simulink model "TestWalsh02_home"  (R2021a)
settings: Solver=VariableStepAuto  StartTime=0.0  StopTime=96  RelTol=1e-3
libraries: dspspect3 x4
settings Model: Creator=alexandr.lanin  LastModifiedBy=Alex
settings SolverCC: AlgebraicLoopSolver=TrustRegion
settings DataIOCC: ReturnWorkspaceOutputs=off
settings DebuggingCC: SFMachineParentedDataDiag=warning  ArithmeticOperatorsInVariantConditions=warning
settings SFSimCC: SimUseLocalCustomCode=off  CustomCodeUndefinedFunction=UseInterfaceOnly
settings RTWCC: RTWUseLocalCustomCode=off
settings CodeAppCC: StateflowObjectComments=on

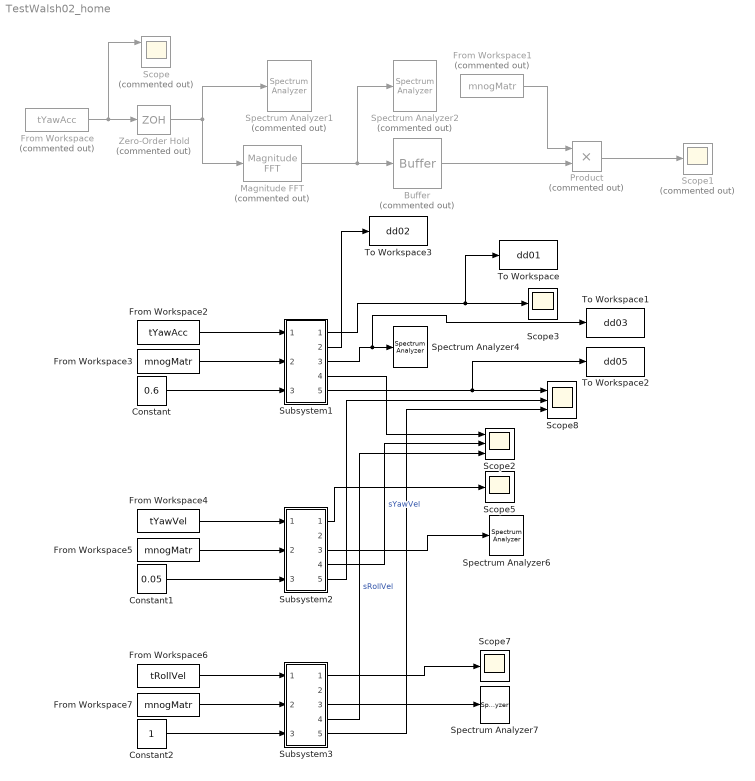
== system TestWalsh02_home ==
  Buffer : Buffer  Commented=on  OutputFrames=off
  Constant : Constant  Value=0.6
  Constant1 : Constant  Value=0.05
  Constant2 : Constant
  From Workspace : FromWorkspace  Commented=on  VariableName=tYawAcc
  From Workspace1 : FromWorkspace  Commented=on  VariableName=mnogMatr
  From Workspace2 : FromWorkspace  VariableName=tYawAcc
  From Workspace3 : FromWorkspace  VariableName=mnogMatr
  From Workspace4 : FromWorkspace  VariableName=tYawVel
  From Workspace5 : FromWorkspace  VariableName=mnogMatr
  From Workspace6 : FromWorkspace  VariableName=tRollVel
  From Workspace7 : FromWorkspace  VariableName=mnogMatr
  Magnitude FFT : dspspect3/Magnitude FFT  Commented=on  mag_or_magsq=Magnitude squared  FFTImplementation=Auto  fftLenInherit=off  fftsize=64  WrapInput=on
      settings: SourceProductBaseCode=DS
  Product : Product  Commented=on
  Scope : Scope  Commented=on  NumInputPorts=3
  Scope1 : Scope  Commented=on
  Scope2 : Scope  NumInputPorts=3
  Scope3 : Scope
  Scope5 : Scope
  Scope7 : Scope
  Scope8 : Scope  NumInputPorts=3
  Spectrum Analyzer1 : SpectrumAnalyzer  Commented=on
  Spectrum Analyzer2 : SpectrumAnalyzer  Commented=on
  Spectrum Analyzer4 : SpectrumAnalyzer
  Spectrum Analyzer6 : SpectrumAnalyzer
  Spectrum Analyzer7 : SpectrumAnalyzer
  Subsystem1 : Subsystem
  Subsystem2 : Subsystem
  Subsystem3 : Subsystem
  To Workspace : ToWorkspace  VariableName=dd01  SaveFormat=Timeseries  SampleTime=-1
  To Workspace1 : ToWorkspace  VariableName=dd03  SaveFormat=Timeseries  SampleTime=-1
  To Workspace2 : ToWorkspace  VariableName=dd05  SaveFormat=Timeseries  SampleTime=-1
  To Workspace3 : ToWorkspace  VariableName=dd02  SaveFormat=Timeseries  SampleTime=-1
  Zero-Order Hold : ZeroOrderHold  Commented=on  SampleTime=0.01
  wires:
  From Workspace/1 -> Zero-Order Hold/1, Scope/1
  Magnitude FFT/1 -> Buffer/1, Spectrum Analyzer2/1
  Zero-Order Hold/1 -> Magnitude FFT/1, Spectrum Analyzer1/1
  Buffer/1 -> Product/2
  From Workspace1/1 -> Product/1
  Product/1 -> Scope1/1
  From Workspace3/1 -> Subsystem1/2(In2)
  From Workspace2/1 -> Subsystem1/1(In1)
  Subsystem1/3(Out3) -> To Workspace1/1, Spectrum Analyzer4/1
  Subsystem1/1(Out1) -> To Workspace/1, Scope3/1
  Subsystem1/4(Out4) -> Scope2/1
  Subsystem2/1(Out1) -> Scope5/1
  Subsystem2/3(Out3) -> Spectrum Analyzer6/1
  From Workspace4/1 -> Subsystem2/1(In1)
  From Workspace5/1 -> Subsystem2/2(In2)
  Subsystem3/4(Out4) -> Scope2/3  "sRollVel"
  Subsystem3/1(Out1) -> Scope7/1
  From Workspace6/1 -> Subsystem3/1(In1)
  Subsystem3/3(Out3) -> Spectrum Analyzer7/1
  From Workspace7/1 -> Subsystem3/2(In3)
  Constant/1 -> Subsystem1/3(In3)
  Constant1/1 -> Subsystem2/3(In3)
  Constant2/1 -> Subsystem3/3(In2)
  Subsystem2/4(Out4) -> Scope2/2  "sYawVel"
  Subsystem3/5(Out5) -> Scope8/3
  Subsystem2/5(Out5) -> Scope8/2
  Subsystem1/5(Out5) -> To Workspace2/1, Scope8/1
  Subsystem1/2(Out2) -> To Workspace3/1

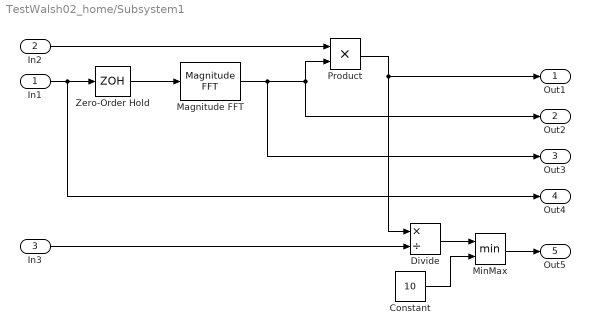
== system TestWalsh02_home/Subsystem1 ==
  In1 : Inport
  In2 : Inport  Port=2
  In3 : Inport  Port=3
  Constant : Constant  Value=10
  Divide : Product  Inputs=*/
  Magnitude FFT : dspspect3/Magnitude FFT  mag_or_magsq=Magnitude squared  FFTImplementation=Auto  fftLenInherit=off  fftsize=64  WrapInput=on
      settings: SourceProductBaseCode=DS
  MinMax : MinMax  Inputs=2
  Product : Product
  Zero-Order Hold : ZeroOrderHold  SampleTime=0.01
  Out1 : Outport
  Out2 : Outport  Port=2
  Out3 : Outport  Port=3
  Out4 : Outport  Port=4
  Out5 : Outport  Port=5
  wires:
  Zero-Order Hold/1 -> Magnitude FFT/1
  In1/1 -> Out4/1, Zero-Order Hold/1
  In2/1 -> Product/1
  In3/1 -> Divide/2
  Divide/1 -> MinMax/1
  Constant/1 -> MinMax/2
  MinMax/1 -> Out5/1
  Product/1 -> Divide/1, Out1/1
  Magnitude FFT/1 -> Out2/1, Product/2, Out3/1

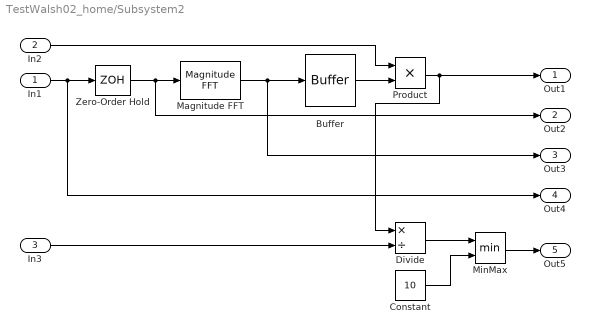
== system TestWalsh02_home/Subsystem2 ==
  In1 : Inport
  In2 : Inport  Port=2
  In3 : Inport  Port=3
  Buffer : Buffer  OutputFrames=off
  Constant : Constant  Value=10
  Divide : Product  Inputs=*/
  Magnitude FFT : dspspect3/Magnitude FFT  mag_or_magsq=Magnitude squared  FFTImplementation=Auto  fftLenInherit=off  fftsize=64  WrapInput=on
      settings: SourceProductBaseCode=DS
  MinMax : MinMax  Inputs=2
  Product : Product
  Zero-Order Hold : ZeroOrderHold  SampleTime=0.01
  Out1 : Outport
  Out2 : Outport  Port=2
  Out3 : Outport  Port=3
  Out4 : Outport  Port=4
  Out5 : Outport  Port=5
  wires:
  Zero-Order Hold/1 -> Out2/1, Magnitude FFT/1
  In1/1 -> Out4/1, Zero-Order Hold/1
  Magnitude FFT/1 -> Out3/1, Buffer/1
  Buffer/1 -> Product/2
  Product/1 -> Divide/1, Out1/1
  In2/1 -> Product/1
  In3/1 -> Divide/2
  Divide/1 -> MinMax/1
  Constant/1 -> MinMax/2
  MinMax/1 -> Out5/1

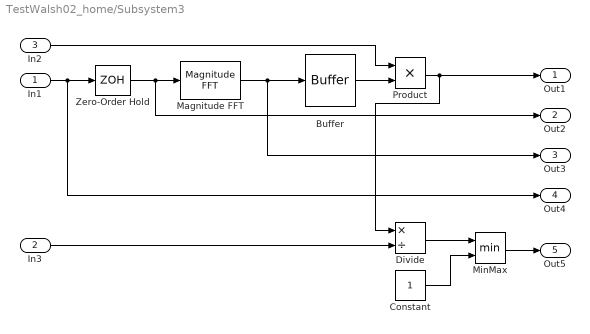
== system TestWalsh02_home/Subsystem3 ==
  In1 : Inport
  In3 : Inport  Port=2
  In2 : Inport  Port=3
  Buffer : Buffer  OutputFrames=off
  Constant : Constant
  Divide : Product  Inputs=*/
  Magnitude FFT : dspspect3/Magnitude FFT  mag_or_magsq=Magnitude squared  FFTImplementation=Auto  fftLenInherit=off  fftsize=64  WrapInput=on
      settings: SourceProductBaseCode=DS
  MinMax : MinMax  Inputs=2
  Product : Product
  Zero-Order Hold : ZeroOrderHold  SampleTime=0.01
  Out1 : Outport
  Out2 : Outport  Port=2
  Out3 : Outport  Port=3
  Out4 : Outport  Port=4
  Out5 : Outport  Port=5
  wires:
  Zero-Order Hold/1 -> Out2/1, Magnitude FFT/1
  In1/1 -> Out4/1, Zero-Order Hold/1
  Magnitude FFT/1 -> Out3/1, Buffer/1
  Buffer/1 -> Product/2
  Product/1 -> Divide/1, Out1/1
  In2/1 -> Product/1
  In3/1 -> Divide/2
  Divide/1 -> MinMax/1
  Constant/1 -> MinMax/2
  MinMax/1 -> Out5/1
